simulink library "Storage_Type_4_CONF"  (Simulink 8.2)
settings: Solver=ode45  StartTime=0.0  StopTime=10.0  RelTol=1e-3
libraries: carnot x2
settings Model: Creator=lena.frank  LastModifiedBy=drhf

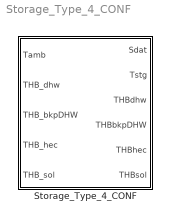
== system Storage_Type_4_CONF ==
  Storage_Type_4_CONF : Subsystem  mask(Combi-storage for hot water production and heating){parameterfile=Default_Storage, tini=[10:5:55]}
      mask prompts: parameterfile "Storage parameter set"; tini "initial temperature (vector or scalar) in °C"
      mask help: Predefinded combi-storage for hot water production and heating configurated to preheat the return of the backup heater.
      mask init:
      | % callback to set parameters of model
      | CarnotCallbacks_StorageConf(4,parameterfile);
      mask Help: web(fullfile(path_carnot('help'),'Storage_Type_N.html'),'-helpbrowser')
      mask TypeOptions parameterfile: Default_Storage
      mask Display:
      | % user defined picture file
      | picfile = fullfile(path_carnot('intlibsl'), ...
      |         'Storage','Thermal','Storage_Type_4_CONF','parameter_set', ...
      |         'Storage_Type_4_CONF.jpg');
      | 
      | % show public picture
      | plot([36,36,40,50,54,54,50,40,36]/100,[90,50,45,45,50,90,93,93,90]/100, ...
      |     [36,51,40,51,36]/100,[50,50,68,85,85]/100,[36,51,44,51,36]/100, ...
      |     [54,54,56,58,58]/100)
      | 
      | % show internal picture if defined
      | if  ~BlockIsInCarnotLibrary       % if not located in library
      |     if exist(picfile)
      |         image(imread(picfile), [0.3, 0, 0.45, 1])
      |         set_param(gcb, 'BackgroundColor', 'White')
      |     end
      | end

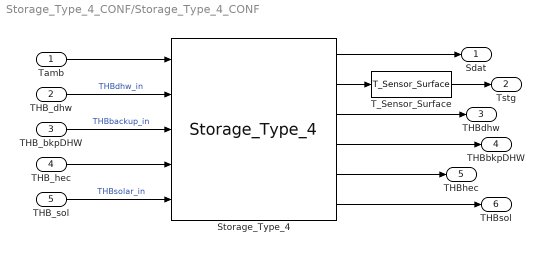
== system Storage_Type_4_CONF/Storage_Type_4_CONF ==
  Tamb : Inport
  THB_dhw : Inport  Port=2
  THB_bkpDHW : Inport  Port=3
  THB_hec : Inport  Port=4
  THB_sol : Inport  Port=5
  Storage_Type_4 : carnot/Storage/Thermal/Storage_Type_4  uloss=0.74  ubot=1.37  utop=0.74  cond=0.62  t0=tini  volume=0.75  dia=0.79  pos=standing cylinder  nconnect=4  nodes=50  mpoints=50
  T_Sensor_Surface : carnot/Control/T_Sensor_Surface  pos="[0.2         0.5         0.6]"  tdel=10  t0=tini(1)
  Sdat : Outport
  Tstg : Outport  Port=2
  THBdhw : Outport  Port=3
  THBbkpDHW : Outport  Port=4
  THBhec : Outport  Port=5
  THBsol : Outport  Port=6
  wires:
  T_Sensor_Surface/1 -> Tstg/1
  THB_hec/1 -> Storage_Type_4/4
  Storage_Type_4/5 -> THBhec/1
  Storage_Type_4/6 -> THBsol/1
  Storage_Type_4/4 -> THBbkpDHW/1
  Storage_Type_4/3 -> THBdhw/1
  Tamb/1 -> Storage_Type_4/1
  THB_dhw/1 -> Storage_Type_4/2  "THBdhw_in"
  THB_bkpDHW/1 -> Storage_Type_4/3  "THBbackup_in"
  THB_sol/1 -> Storage_Type_4/5  "THBsolar_in"
  Storage_Type_4/1 -> Sdat/1
  Storage_Type_4/2 -> T_Sensor_Surface/1
